simulink model "PoseEstimationController"  (R2017a)
settings: Solver=FixedStepDiscrete  StartTime=0.0  StopTime=10.0  RelTol=1e-3
values from neighbouring files (symbols this model uses):
  dt = dtFC    [evalOriginSensordata.m]    (also in startControllerNL.m = 0.01)
  H_Drone = zeros(5,12)    [evalOriginSensordata.m]    (also in startControllerNL.m)
  H_TWB = zeros(3,12)    [evalOriginSensordata.m]    (also in startControllerNL.m)
  k1 = a    (= 1)    [evalOriginSensordata.m]    (also in startControllerNL.m)
  k10 = a    (= 1)    [evalOriginSensordata.m]    (also in startControllerNL.m)
  k11 = a    (= 1)    [evalOriginSensordata.m]    (also in startControllerNL.m)
  k12 = a    (= 1)    [evalOriginSensordata.m]    (also in startControllerNL.m)
  k2 = a    (= 1)    [evalOriginSensordata.m]    (also in startControllerNL.m)
  k3 = a    (= 1)    [evalOriginSensordata.m]    (also in startControllerNL.m)
  k4 = a    (= 1)    [evalOriginSensordata.m]    (also in startControllerNL.m)
  k5 = a    (= 1)    [evalOriginSensordata.m]    (also in startControllerNL.m)
  k6 = a    (= 1)    [evalOriginSensordata.m]    (also in startControllerNL.m)
  k7 = a    (= 1)    [evalOriginSensordata.m]    (also in startControllerNL.m)
  k8 = a    (= 1)    [evalOriginSensordata.m]    (also in startControllerNL.m)
  k9 = a    (= 1)    [evalOriginSensordata.m]    (also in startControllerNL.m)
  kd1 = d    (= 10)    [evalOriginSensordata.m]    (also in startControllerNL.m)
  kd2 = d    (= 10)    [evalOriginSensordata.m]    (also in startControllerNL.m)
  kd3 = d    (= 10)    [evalOriginSensordata.m]    (also in startControllerNL.m)
  kd4 = d    (= 10)    [evalOriginSensordata.m]    (also in startControllerNL.m)
  kp1 = p    (= 5)    [evalOriginSensordata.m]    (also in startControllerNL.m)
  kp2 = p    (= 5)    [evalOriginSensordata.m]    (also in startControllerNL.m)
  kp3 = p    (= 5)    [evalOriginSensordata.m]    (also in startControllerNL.m)
  kp4 = p    (= 5)    [evalOriginSensordata.m]    (also in startControllerNL.m)
libraries: sharedTrackingLibrary x1
settings Model: Creator=Schalker  LastModifiedBy=Schalker
settings OptimizationCC: DefaultParameterBehavior=Inlined  UseDivisionForNetSlopeComputation=on  UseFloatMulNetSlope=on  InlineInvariantSignals=on  PassReuseOutputArgsAs=Individual arguments  ZeroExternalMemoryAtStartup=off  ZeroInternalMemoryAtStartup=off  NoFixptDivByZeroProtection=on  EfficientFloat2IntCast=on  LifeSpan=1  MaxStackSize=64
settings DebuggingCC: ParameterTunabilityLossMsg=error
settings HardwareCC: ProdBitPerPointer=32  ProdBitPerSizeT=32  ProdBitPerPtrDiffT=32  ProdLargestAtomicFloat=None  ProdWordSize=32  ProdHWDeviceType=Custom Processor->Custom
settings SFSimCC: MATLABDynamicMemAlloc=off
settings RTWCC: SystemTargetFile=ert.tlc  GenCodeOnly=on  TemplateMakefile=ert_default_tmf  Description=Embedded Coder  GenerateReport=on  Toolchain=Microsoft Visual C++ 2015 v14.0 | nmake (64-bit Windows)  IncludeHyperlinkInReport=on  LaunchReport=on  TargetLang=C++  GenerateTraceInfo=on  GenerateTraceReport=on  GenerateTraceReportSl=on  GenerateTraceReportSf=on  GenerateTraceReportEml=on  GenerateCodeMetricsReport=on
settings CodeAppCC: ForceParamTrailComments=on  IgnoreCustomStorageClasses=off  OperatorAnnotations=on  SimulinkDataObjDesc=on  SFDataObjDesc=on  MATLABFcnDesc=on  CustomSymbolStrGlobalVar=rt$N$M  CustomSymbolStrType=$N$M  CustomSymbolStrFcn=$N$M$F  CustomSymbolStrMacro=$N$M  InsertBlockDesc=on  MATLABSourceComments=on
settings ERTTargetCC: TargetLangStandard=C++03 (ISO)  IncludeMdlTerminateFcn=off  CombineSignalStateStructs=on  SupportAbsoluteTime=off  SupportComplex=off  SupportNonInlinedSFcns=on  InlinedParameterPlacement=NonHierarchical  RootIOFormat=Structure reference  ERTCustomFileTemplate=example_file_process.tlc  ERTFilePackagingFormat=CompactWithDataFile

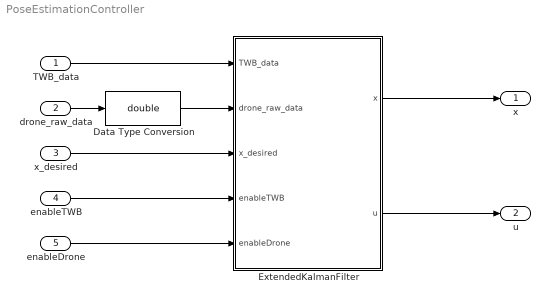
== system PoseEstimationController ==
  "TWB_data " : Inport  OutDataTypeStr=double  PortDimensions=3
  drone_raw_data : Inport  Port=2  OutDataTypeStr=uint8  PortDimensions=11
  x_desired : Inport  Port=3  OutDataTypeStr=double  PortDimensions=4
  enableTWB : Inport  Port=4  OutDataTypeStr=boolean  PortDimensions=1
  enableDrone : Inport  Port=5  OutDataTypeStr=boolean  PortDimensions=1
  Data Type Conversion : DataTypeConversion  OutDataTypeStr=double
  "ExtendedKalmanFilter " : Subsystem  InitFcn=|
      | t_end = 10;
      | Ts = 1/100; %0.05;
      | dt = 1/100;
      | 
      | k1 = 0.5;
      | k2 = 0.5;
      | k3 = 0.5;
      | k4 = 0.5;
      | k5 = 0.5;
      | k6 = 0.5;
      | k7 = 0.5;
      | k8 = 0.5;
      | k9 = 0.5;
      | k10 = 0.5;
      | k11 = 0.5;
      | k12 = 0.5;
      | 
      | a = 1;
      | k1 = a;
      | k2 = a;
      | k3 = a;
      | k4 = a;
      | k5 = a;
      | k6 = a;
      | k7 = a;
      | k8 = a;
      | k9 = a;
      | k10 = a;
      | k11 = a;
      | k12 = a;
      | 
      | p = 5;
      | kp1 = p;
      | kp2 = p;
      | kp3 = p;
      | kp4 = p;
      | 
      | d = 10;
      | kd1 = d;
      | kd2 = d;
      | kd3 = d;
      | kd4 = d;
      | 
      | processNoiseCovariance = eye(12,12)*0.5;
      | measurementNoiseCovarianceTWB = [0.000114037489420717 -2.82089891064414e-06 1.40417613824518e-05;-2.82089891064414e-06 0.000115657032079071 1.08946618253263e-06;1.40417613824518e-05 1.08946618253263e-06 0.00137780347424666];
      | measurementNoiseCovarianceDrone = [7.40493968128454e-07 4.00871171116695e-08 2.64850251168023e-07 4.81776544321576e-08 1.70610840898493e-07;4.00871171116695e-08 1.12410457478521e-06 -8.65404287048207e-08 -1.99569229909733e-07 2.12891815399967e-07;2.64850251168023e-07 -8.65404287048207e-08 3.89370394407336e-05 -1.56813743542319e-06 -2.34614557587901e-06;4.81776544321576e-08 -1.99569229909733e-07 -1.56813743542319e-06 3.83263259074627e-05 1.99513110891507e-06;1.70610840898493e-07 2.12891815399967e-07 -2.34614557587901e-06 1.99513110891507e-06 2.60130783647397e-05];
      | H_TWB = zeros(3,12);
      | H_TWB(1,1) = 1;
      | H_TWB(2,2) = 1;
      | H_TWB(3,3) = 1;
      | 
      | H_Drone = zeros(5,12);
      | H_Drone(1,7) = 1;
      | H_Drone(2,8) = 1;
      | H_Drone(3,9) = 1;
      | H_Drone(4,10) = 1;
      | H_Drone(5,11) = 1;
  x : Outport
  u : Outport  Port=2  OutDataTypeStr=uint8
  wires:
  drone_raw_data/1 -> Data Type Conversion/1
  x_desired/1 -> "ExtendedKalmanFilter "/3(x_desired)
  "ExtendedKalmanFilter "/1(x) -> x/1
  "ExtendedKalmanFilter "/2(u) -> u/1
  Data Type Conversion/1 -> "ExtendedKalmanFilter "/2(drone_raw_data)
  "TWB_data "/1 -> "ExtendedKalmanFilter "/1(TWB_data)
  enableTWB/1 -> "ExtendedKalmanFilter "/4(enableTWB)
  enableDrone/1 -> "ExtendedKalmanFilter "/5(enableDrone)

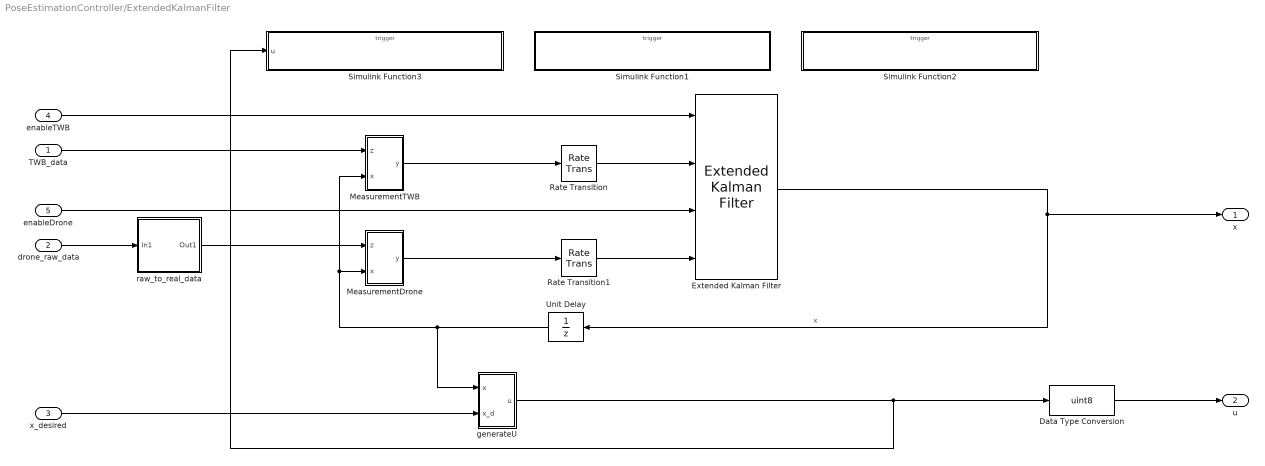
== system PoseEstimationController/ExtendedKalmanFilter  ==
  TWB_data : Inport
  drone_raw_data : Inport  Port=2
  x_desired : Inport  Port=3
  enableTWB : Inport  Port=4
  enableDrone : Inport  Port=5
  Data Type Conversion : DataTypeConversion  OutDataTypeStr=uint8
  Extended Kalman Filter : sharedTrackingLibrary/Extended Kalman Filter  StateTransitionFcn=stateTransitionFcn  HasStateTransitionJacobianFcn=off  HasAdditiveProcessNoise=Additive  ProcessNoise=processNoiseCovariance  HasTimeVaryingProcessNoise=off  HasStateTransitionFcnExtraArgument=0  InitialState=zeros(12, 1)  InitialStateCovariance=10  MeasurementFcn1=measurementTWBFcn  HasMeasurementJacobianFcn1=off  HasMeasurementEnablePort1=on  HasAdditiveMeasurementNoise1=Additive  MeasurementNoise1=measurementNoiseCovarianceTWB  HasTimeVaryingMeasurementNoise1=off  HasMeasurementFcnExtraArgument1=0  MeasurementFcn2=measurementDroneFcn  HasMeasurementJacobianFcn2=off  HasMeasurementEnablePort2=on  HasAdditiveMeasurementNoise2=Additive  MeasurementNoise2=measurementNoiseCovarianceDrone  HasTimeVaryingMeasurementNoise2=off  HasMeasurementFcnExtraArgument2=0  MeasurementFcn3=myMeasurementFcn  HasMeasurementJacobianFcn3=off  HasMeasurementEnablePort3=off  HasAdditiveMeasurementNoise3=Additive  MeasurementNoise3=1  HasTimeVaryingMeasurementNoise3=off  HasMeasurementFcnExtraArgument3=0  MeasurementFcn4=myMeasurementFcn  HasMeasurementJacobianFcn4=off  HasMeasurementEnablePort4=off  HasAdditiveMeasurementNoise4=Additive  MeasurementNoise4=1  HasTimeVaryingMeasurementNoise4=off  HasMeasurementFcnExtraArgument4=0  MeasurementFcn5=myMeasurementFcn  HasMeasurementJacobianFcn5=off  HasMeasurementEnablePort5=off  HasAdditiveMeasurementNoise5=Additive  MeasurementNoise5=1  HasTimeVaryingMeasurementNoise5=off  HasMeasurementFcnExtraArgument5=0  EnableMultirate=on  StateTransitionFcnSampleTime=dt  MeasurementFcn1SampleTime=dt  MeasurementFcn2SampleTime=dt  MeasurementFcn3SampleTime=1  MeasurementFcn4SampleTime=1  MeasurementFcn5SampleTime=1  UseCurrentEstimator=on  OutputStateCovariance=off  DataType=double  SampleTime=1  NumberOfMeasurements=2
  MeasurementDrone : Subsystem
  MeasurementTWB : Subsystem
  Rate Transition : RateTransition
  Rate Transition1 : RateTransition
  Simulink Function1 : Subsystem  TreatAsAtomicUnit=on
  Simulink Function2 : Subsystem  TreatAsAtomicUnit=on
  Simulink Function3 : Subsystem  TreatAsAtomicUnit=on
  Unit Delay : UnitDelay  SampleTime=-1
  generateU : Subsystem
  raw_to_real_data : Subsystem
  x : Outport
  u : Outport  Port=2
  wires:
  TWB_data/1 -> MeasurementTWB/1(z)
  x_desired/1 -> generateU/2("x_d ")
  Extended Kalman Filter/1 -> Unit Delay/1, x/1  "x"
  MeasurementDrone/1(y) -> Rate Transition1/1
  Rate Transition1/1 -> Extended Kalman Filter/4
  drone_raw_data/1 -> raw_to_real_data/1(In1)
  Rate Transition/1 -> Extended Kalman Filter/2
  Unit Delay/1 -> MeasurementDrone/2(x), MeasurementTWB/2(x), generateU/1(x)
  generateU/1(u) -> Data Type Conversion/1, Simulink Function3/1(u)
  MeasurementTWB/1(y) -> Rate Transition/1
  raw_to_real_data/1(Out1) -> MeasurementDrone/1(z)
  Data Type Conversion/1 -> u/1
  enableTWB/1 -> Extended Kalman Filter/1
  enableDrone/1 -> Extended Kalman Filter/3

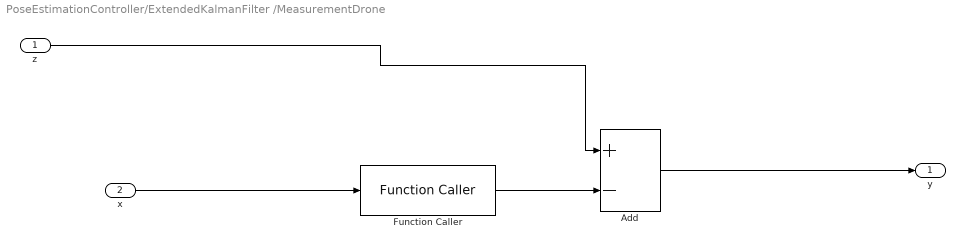
== system PoseEstimationController/ExtendedKalmanFilter /MeasurementDrone ==
  z : Inport
  x : Inport  Port=2
  Add : Sum  Inputs=+-
  Function Caller : FunctionCaller  FunctionPrototype=y = measurementDroneFcn(x)
  y : Outport
  wires:
  Add/1 -> y/1
  z/1 -> Add/1
  Function Caller/1 -> Add/2
  x/1 -> Function Caller/1

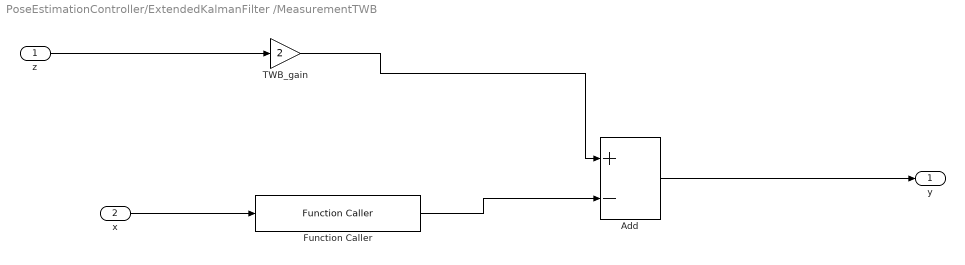
== system PoseEstimationController/ExtendedKalmanFilter /MeasurementTWB ==
  z : Inport
  x : Inport  Port=2
  Add : Sum  Inputs=+-
  Function Caller : FunctionCaller  FunctionPrototype=y = measurementTWBFcn(x)
  TWB_gain : Gain  Gain=2
  y : Outport
  wires:
  z/1 -> TWB_gain/1
  Add/1 -> y/1
  Function Caller/1 -> Add/2
  x/1 -> Function Caller/1
  TWB_gain/1 -> Add/1

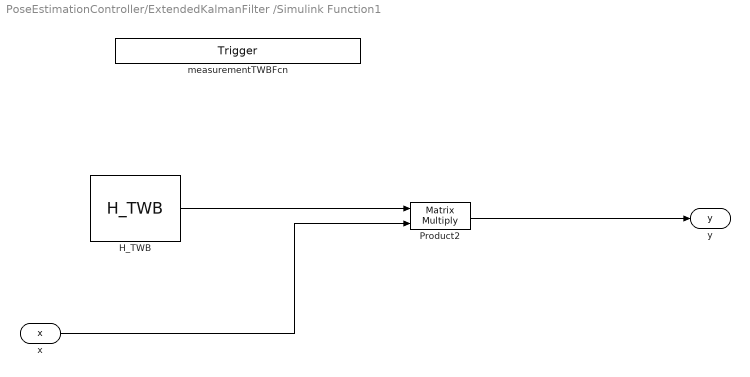
== system PoseEstimationController/ExtendedKalmanFilter /Simulink Function1 ==
  measurementTWBFcn : TriggerPort  TriggerType=function-call  IsSimulinkFunction=on  FunctionName=measurementTWBFcn  VariantControl=Variant
  H_TWB : Constant  Value=H_TWB
  Product2 : Product  Multiplication=Matrix(*)
  x : ArgIn  DisableCoverage=on  PortDimensions=12  ArgumentName=x
  y : ArgOut  DisableCoverage=on  PortDimensions=3  ArgumentName=y
  wires:
  H_TWB/1 -> Product2/1
  x/1 -> Product2/2
  Product2/1 -> y/1

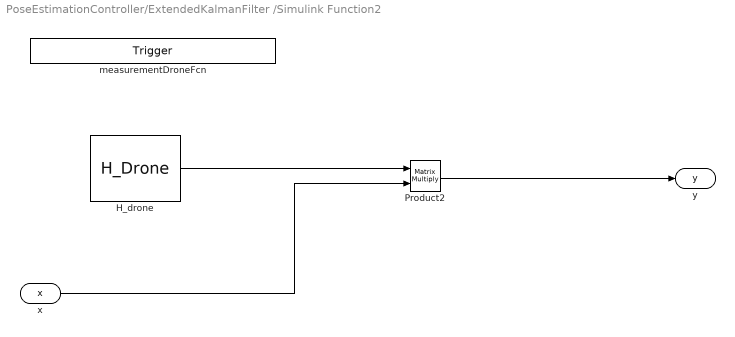
== system PoseEstimationController/ExtendedKalmanFilter /Simulink Function2 ==
  measurementDroneFcn : TriggerPort  TriggerType=function-call  IsSimulinkFunction=on  FunctionName=measurementDroneFcn  VariantControl=Variant
  H_drone : Constant  Value=H_Drone
  Product2 : Product  Multiplication=Matrix(*)
  x : ArgIn  DisableCoverage=on  PortDimensions=12  ArgumentName=x
  y : ArgOut  DisableCoverage=on  PortDimensions=5  ArgumentName=y
  wires:
  Product2/1 -> y/1
  H_drone/1 -> Product2/1
  x/1 -> Product2/2

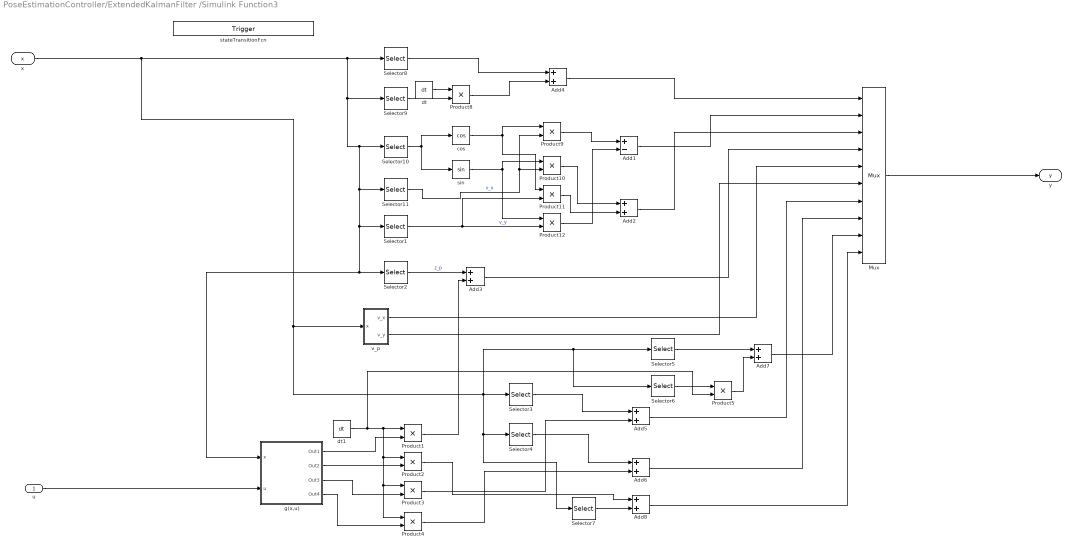
== system PoseEstimationController/ExtendedKalmanFilter /Simulink Function3 ==
  u : Inport
  stateTransitionFcn : TriggerPort  TriggerType=function-call  IsSimulinkFunction=on  FunctionName=stateTransitionFcn  VariantControl=Variant
  Add1 : Sum  Inputs=+-
  Add{2..8} (7 alike) : Sum
  Mux : Mux  Inputs=10
  Product{1..5,8..12} (10 alike) : Product
  Selector1 : Selector  InputPortWidth=12  IndexOptions=Index vector (dialog)  Indices=[8]  OutputSizes=1
  Selector10 : Selector  InputPortWidth=12  IndexOptions=Index vector (dialog)  Indices=[11]  OutputSizes=1
  Selector11 : Selector  InputPortWidth=12  IndexOptions=Index vector (dialog)  Indices=[7]  OutputSizes=1
  Selector2 : Selector  InputPortWidth=12  IndexOptions=Index vector (dialog)  Indices=[6]  OutputSizes=1
  Selector3 : Selector  InputPortWidth=12  IndexOptions=Index vector (dialog)  Indices=[9]  OutputSizes=1
  Selector4 : Selector  InputPortWidth=12  IndexOptions=Index vector (dialog)  Indices=[10]  OutputSizes=1
  Selector5 : Selector  InputPortWidth=12  IndexOptions=Index vector (dialog)  Indices=[11]  OutputSizes=1
  Selector6 : Selector  InputPortWidth=12  IndexOptions=Index vector (dialog)  Indices=[12]  OutputSizes=1
  Selector7 : Selector  InputPortWidth=12  IndexOptions=Index vector (dialog)  Indices=[12]  OutputSizes=1
  Selector8 : Selector  InputPortWidth=12  IndexOptions=Index vector (dialog)  Indices=[1 2 3]  OutputSizes=1
  Selector9 : Selector  InputPortWidth=12  IndexOptions=Index vector (dialog)  Indices=[4 5 6]  OutputSizes=1
  cos : Trigonometry  Operator=cos
  dt : Constant  Value=dt
  dt1 : Constant  Value=dt
  g(x,u) : Subsystem
  sin : Trigonometry
  v_p : Subsystem
  x : ArgIn  DisableCoverage=on  PortDimensions=12  ArgumentName=x
  y : ArgOut  DisableCoverage=on  PortDimensions=12  ArgumentName=y
  wires:
  x/1 -> Selector6/1, Selector5/1, Selector7/1, Selector4/1, Selector3/1, v_p/1(x), Selector8/1, Selector11/1, Selector1/1, Selector2/1, g(x,u)/1(x), Selector10/1, Selector9/1
  Selector9/1 -> Product8/2
  dt/1 -> Product8/1
  Product8/1 -> Add4/2
  Selector8/1 -> Add4/1
  Add4/1 -> Mux/1
  Selector10/1 -> sin/1, cos/1
  cos/1 -> Product11/1, Product9/1
  sin/1 -> Product12/1, Product10/1
  u/1 -> g(x,u)/2(u)
  Selector11/1 -> Product10/2, Product9/2  "v_x"
  Selector1/1 -> Product12/2, Product11/2  "v_y"
  Product9/1 -> Add1/1
  Product12/1 -> Add1/2
  Product10/1 -> Add2/1
  Product11/1 -> Add2/2
  Selector2/1 -> Add3/1  "z_p"
  g(x,u)/1(Out1) -> Product1/2
  Product1/1 -> Add3/2
  g(x,u)/2(Out2) -> Product2/2
  g(x,u)/3(Out3) -> Product3/2
  g(x,u)/4(Out4) -> Product4/2
  Add3/1 -> Mux/4
  v_p/1(v_x) -> Mux/5
  v_p/2(v_y) -> Mux/6
  Add1/1 -> Mux/2
  Add2/1 -> Mux/3
  Selector3/1 -> Add5/1
  Product3/1 -> Add5/2
  Selector4/1 -> Add6/1
  Product4/1 -> Add6/2
  Add5/1 -> Mux/7
  Add6/1 -> Mux/8
  Selector6/1 -> Product5/1
  dt1/1 -> Product5/2, Product2/1, Product4/1, Product3/1, Product1/1
  Selector5/1 -> Add7/1
  Product5/1 -> Add7/2
  Add7/1 -> Mux/9
  Selector7/1 -> Add8/2
  Product2/1 -> Add8/1
  Add8/1 -> Mux/10
  Mux/1 -> y/1

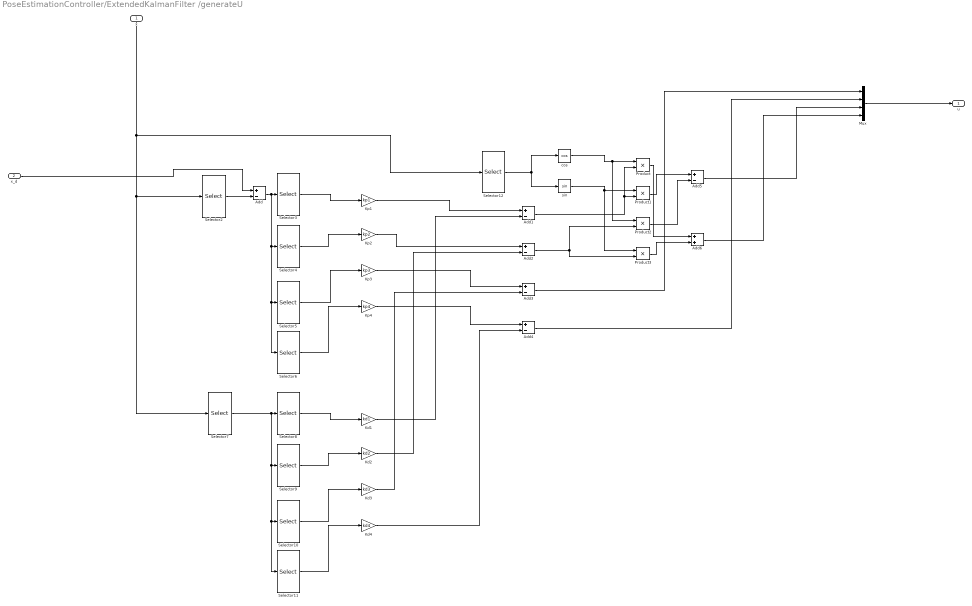
== system PoseEstimationController/ExtendedKalmanFilter /generateU ==
  x : Inport
  "x_d " : Inport  Port=2
  Add{,1..5} (6 alike) : Sum  Inputs=+-
  Add6 : Sum
  Kd1 : Gain  Gain=kd1
  Kd2 : Gain  Gain=kd2
  Kd3 : Gain  Gain=kd3
  Kd4 : Gain  Gain=kd4
  Kp1 : Gain  Gain=kp1
  Kp2 : Gain  Gain=kp2
  Kp3 : Gain  Gain=kp3
  Kp4 : Gain  Gain=kp4
  Mux : Mux
  Product{,1..3} (4 alike) : Product
  Selector10 : Selector  InputPortWidth=4  IndexOptions=Index vector (dialog)  Indices=3  OutputSizes=1
  Selector11 : Selector  InputPortWidth=4  IndexOptions=Index vector (dialog)  Indices=4  OutputSizes=1
  Selector12 : Selector  InputPortWidth=12  IndexOptions=Index vector (dialog)  Indices=11  OutputSizes=1
  Selector2 : Selector  InputPortWidth=12  IndexOptions=Index vector (dialog)  Indices=[1 2 3 11]  OutputSizes=1
  Selector3 : Selector  InputPortWidth=4  IndexOptions=Index vector (dialog)  Indices=[1]  OutputSizes=1
  Selector4 : Selector  InputPortWidth=4  IndexOptions=Index vector (dialog)  Indices=2  OutputSizes=1
  Selector5 : Selector  InputPortWidth=4  IndexOptions=Index vector (dialog)  Indices=3  OutputSizes=1
  Selector6 : Selector  InputPortWidth=4  IndexOptions=Index vector (dialog)  Indices=4  OutputSizes=1
  Selector7 : Selector  InputPortWidth=12  IndexOptions=Index vector (dialog)  Indices=[4 5 6 12]  OutputSizes=1
  Selector8 : Selector  InputPortWidth=4  IndexOptions=Index vector (dialog)  Indices=[1]  OutputSizes=1
  Selector9 : Selector  InputPortWidth=4  IndexOptions=Index vector (dialog)  Indices=2  OutputSizes=1
  cos : Trigonometry  Operator=cos
  sin : Trigonometry
  u : Outport
  wires:
  Selector3/1 -> Kp1/1
  "x_d "/1 -> Add/1
  Kp2/1 -> Add2/1
  Product2/1 -> Add5/2
  Add2/1 -> Product3/2, Product2/2
  Selector4/1 -> Kp2/1
  Add4/1 -> Mux/2
  Selector2/1 -> Add/2
  Add6/1 -> Mux/4
  Add5/1 -> Mux/3
  Product1/1 -> Add5/1
  Kp1/1 -> Add1/1
  Selector6/1 -> Kp4/1
  Kd4/1 -> Add4/2
  Add3/1 -> Mux/1
  Selector11/1 -> Kd4/1
  Selector7/1 -> Selector8/1, Selector9/1, Selector10/1, Selector11/1
  Selector10/1 -> Kd3/1
  Selector9/1 -> Kd2/1
  Selector8/1 -> Kd1/1
  Kd3/1 -> Add3/2
  Kp4/1 -> Add4/1
  Add1/1 -> Product1/2, Product/2
  Selector12/1 -> cos/1, sin/1
  Add/1 -> Selector6/1, Selector5/1, Selector4/1, Selector3/1
  Kd1/1 -> Add1/2
  x/1 -> Selector12/1, Selector7/1, Selector2/1
  Kp3/1 -> Add3/1
  Product3/1 -> Add6/2
  Product/1 -> Add6/1
  cos/1 -> Product2/1, Product/1
  sin/1 -> Product3/1, Product1/1
  Kd2/1 -> Add2/2
  Mux/1 -> u/1
  Selector5/1 -> Kp3/1

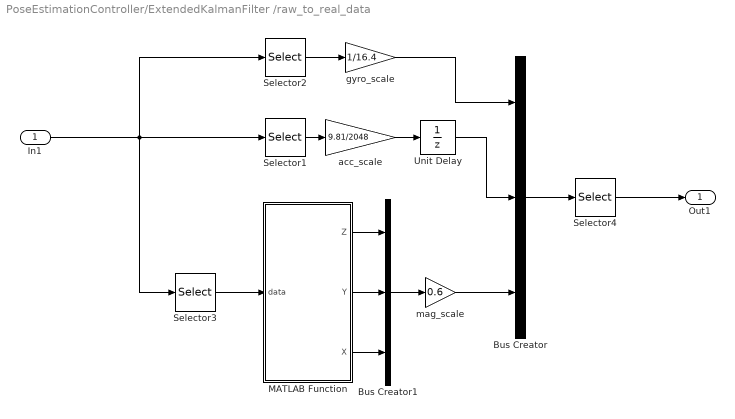
== system PoseEstimationController/ExtendedKalmanFilter /raw_to_real_data ==
  In1 : Inport  PortDimensions=11
  Bus Creator : BusCreator  Inputs=3
  Bus Creator1 : BusCreator  Inputs=3
  MATLAB Function : MATLAB Function  TreatAsAtomicUnit=on
  Selector1 : Selector  InputPortWidth=11  IndexOptions=Index vector (dialog)  Indices=[4,5,6]  OutputSizes=1
  Selector2 : Selector  InputPortWidth=11  IndexOptions=Index vector (dialog)  Indices=[1,2,3]  OutputSizes=1
  Selector3 : Selector  InputPortWidth=11  IndexOptions=Index vector (dialog)  Indices=[1:9]  OutputSizes=1
  Selector4 : Selector  InputPortWidth=9  IndexOptions=Index vector (dialog)  Indices=[4,5,7,8,9]  OutputSizes=1
  Unit Delay : UnitDelay  SampleTime=-1
  acc_scale : Gain  Gain=9.81/2048
  gyro_scale : Gain  Gain=1/16.4
  mag_scale : Gain  Gain=0.6
  Out1 : Outport  PortDimensions=5
  wires:
  In1/1 -> Selector3/1, Selector1/1, Selector2/1
  MATLAB Function/1(Z) -> Bus Creator1/1
  Bus Creator/1 -> Selector4/1
  Selector2/1 -> gyro_scale/1
  Selector1/1 -> acc_scale/1
  gyro_scale/1 -> Bus Creator/1
  Selector3/1 -> MATLAB Function/1(data)
  MATLAB Function/2(Y) -> Bus Creator1/2
  mag_scale/1 -> Bus Creator/3
  MATLAB Function/3(X) -> Bus Creator1/3
  Selector4/1 -> Out1/1
  Bus Creator1/1 -> mag_scale/1
  acc_scale/1 -> Unit Delay/1
  Unit Delay/1 -> Bus Creator/2

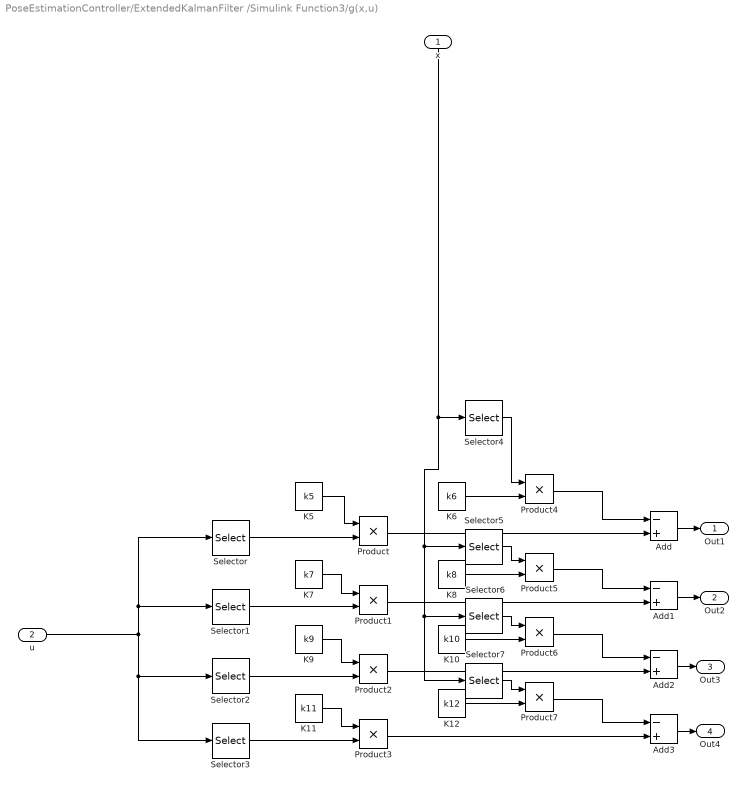
== system PoseEstimationController/ExtendedKalmanFilter /Simulink Function3/g(x,u) ==
  x : Inport
  u : Inport  Port=2
  Add{,1..3} (4 alike) : Sum  Inputs=-+
  K10 : Constant  Value=k10
  K11 : Constant  Value=k11
  K12 : Constant  Value=k12
  K5 : Constant  Value=k5
  K6 : Constant  Value=k6
  K7 : Constant  Value=k7
  K8 : Constant  Value=k8
  K9 : Constant  Value=k9
  Product{,1..7} (8 alike) : Product
  Selector : Selector  InputPortWidth=4  IndexOptions=Index vector (dialog)  Indices=[1]  OutputSizes=1
  Selector1 : Selector  InputPortWidth=4  IndexOptions=Index vector (dialog)  Indices=[2]  OutputSizes=1
  Selector2 : Selector  InputPortWidth=4  IndexOptions=Index vector (dialog)  Indices=[3]  OutputSizes=1
  Selector3 : Selector  InputPortWidth=4  IndexOptions=Index vector (dialog)  Indices=[4]  OutputSizes=1
  Selector4 : Selector  InputPortWidth=12  IndexOptions=Index vector (dialog)  Indices=[6]  OutputSizes=1
  Selector5 : Selector  InputPortWidth=12  IndexOptions=Index vector (dialog)  Indices=[12]  OutputSizes=1
  Selector6 : Selector  InputPortWidth=12  IndexOptions=Index vector (dialog)  Indices=[9]  OutputSizes=1
  Selector7 : Selector  InputPortWidth=12  IndexOptions=Index vector (dialog)  Indices=[10]  OutputSizes=1
  Out1 : Outport
  Out2 : Outport  Port=2
  Out3 : Outport  Port=3
  Out4 : Outport  Port=4
  wires:
  K7/1 -> Product1/1
  Selector6/1 -> Product6/1
  Selector2/1 -> Product2/2
  Product/1 -> Add/2
  Product6/1 -> Add2/1
  Selector/1 -> Product/2
  Add2/1 -> Out3/1
  x/1 -> Selector7/1, Selector6/1, Selector5/1, Selector4/1
  Add3/1 -> Out4/1
  Add/1 -> Out1/1
  Add1/1 -> Out2/1
  K9/1 -> Product2/1
  Selector4/1 -> Product4/1
  u/1 -> Selector/1, Selector1/1, Selector3/1, Selector2/1
  Product2/1 -> Add2/2
  K8/1 -> Product5/2
  Product3/1 -> Add3/2
  Product1/1 -> Add1/2
  Selector5/1 -> Product5/1
  Product5/1 -> Add1/1
  Selector3/1 -> Product3/2
  K5/1 -> Product/1
  K12/1 -> Product7/2
  Product7/1 -> Add3/1
  K10/1 -> Product6/2
  Product4/1 -> Add/1
  Selector1/1 -> Product1/2
  Selector7/1 -> Product7/1
  K11/1 -> Product3/1
  K6/1 -> Product4/2

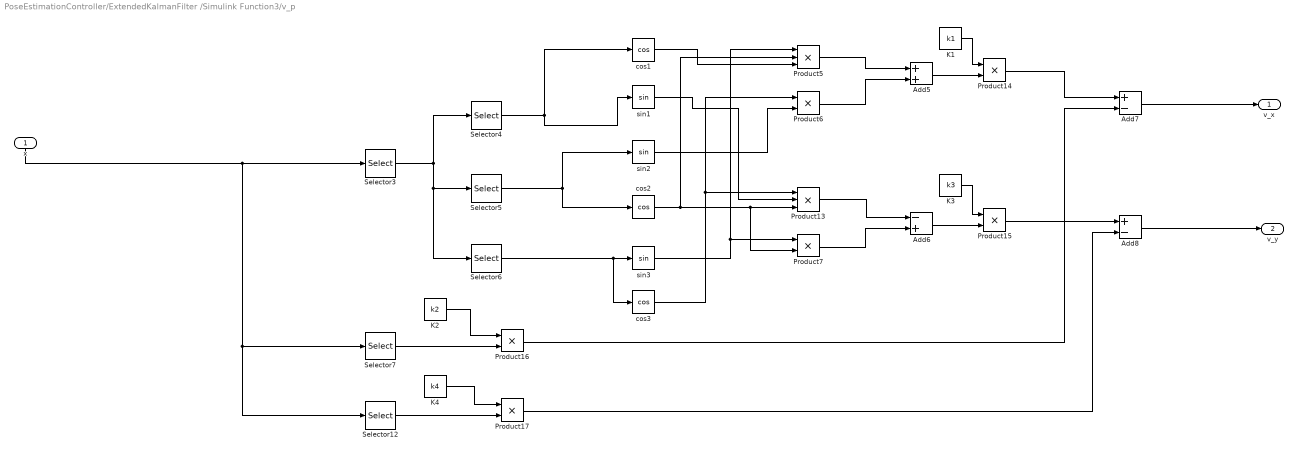
== system PoseEstimationController/ExtendedKalmanFilter /Simulink Function3/v_p ==
  x : Inport
  Add5 : Sum
  Add6 : Sum  Inputs=-+
  Add7 : Sum  Inputs=+-
  Add8 : Sum  Inputs=+-
  K1 : Constant  Value=k1
  K2 : Constant  Value=k2
  K3 : Constant  Value=k3
  K4 : Constant  Value=k4
  Product13 : Product  Inputs=3
  Product{6..7,14..17} (6 alike) : Product
  Product5 : Product  Inputs=3
  Selector12 : Selector  InputPortWidth=12  IndexOptions=Index vector (dialog)  Indices=[8]  OutputSizes=1
  Selector3 : Selector  InputPortWidth=12  IndexOptions=Index vector (dialog)  Indices=[9 10 11]  OutputSizes=1
  Selector4 : Selector  InputPortWidth=3  IndexOptions=Index vector (dialog)  Indices=[1]  OutputSizes=1
  Selector5 : Selector  InputPortWidth=3  IndexOptions=Index vector (dialog)  Indices=[2]  OutputSizes=1
  Selector6 : Selector  InputPortWidth=3  IndexOptions=Index vector (dialog)  Indices=[3]  OutputSizes=1
  Selector7 : Selector  InputPortWidth=12  IndexOptions=Index vector (dialog)  Indices=[7]  OutputSizes=1
  cos1 : Trigonometry  Operator=cos
  cos2 : Trigonometry  Operator=cos
  cos3 : Trigonometry  Operator=cos
  sin1 : Trigonometry
  sin2 : Trigonometry
  sin3 : Trigonometry
  v_x : Outport
  v_y : Outport  Port=2
  wires:
  x/1 -> Selector12/1, Selector7/1, Selector3/1
  Selector6/1 -> sin3/1, cos3/1
  sin2/1 -> Product6/2
  Product6/1 -> Add5/2
  Add7/1 -> v_x/1
  Add5/1 -> Product14/2
  K1/1 -> Product14/1
  Product13/1 -> Add6/1
  Product16/1 -> Add7/2
  Product17/1 -> Add8/2
  cos2/1 -> Product7/2, Product13/3, Product5/2
  K2/1 -> Product16/1
  Selector5/1 -> cos2/1, sin2/1
  sin1/1 -> Product13/2
  Add8/1 -> v_y/1
  Selector7/1 -> Product16/2
  Product14/1 -> Add7/1
  sin3/1 -> Product5/1, Product7/1
  Product5/1 -> Add5/1
  Selector12/1 -> Product17/2
  Selector4/1 -> cos1/1, sin1/1
  Selector3/1 -> Selector6/1, Selector5/1, Selector4/1
  Product7/1 -> Add6/2
  Product15/1 -> Add8/1
  Add6/1 -> Product15/2
  cos3/1 -> Product13/1, Product6/1
  cos1/1 -> Product5/3
  K4/1 -> Product17/1
  K3/1 -> Product15/1

== matlab function PoseEstimationController/ExtendedKalmanFilter /raw_to_real_data/MATLAB Function ==
  data: data input; Z output; Y output; X output
function [Z,Y,X] = fcn(data)
    %% Process sensor data through algorithm
    data = data';
    gyroscope = data(1,[1:3]);
    accelerometer = data(1,[4:6]);
    magnetometer = data(1,[7:9]);
    AHRS = MadgwickAHRS('SamplePeriod', 1/256, 'Beta', 0.1);
    % AHRS = MahonyAHRS('SamplePeriod', 1/256, 'Kp', 0.5);

    quaternion = zeros(1, 4);
    AHRS.Update(gyroscope(1,:) * (pi/180), accelerometer(1,:), magnetometer(1,:));	% gyroscope units must be radians
    quaternion = AHRS.Quaternion;

    euler = quatern2euler(quaternConj(quaternion)) * (180/pi);	% use conjugate for sensor frame relative to Earth and convert to degrees.
    Z = euler(1,1);
    Y = euler(1,2);
    X = euler(1,3);

end

% function obj = MadgwickAHRS(varargin)
%     for i = 1:2:nargin
%         if  strcmp(varargin{i}, 'SamplePeriod'), obj.SamplePeriod = varargin{i+1};
%         elseif  strcmp(varargin{i}, 'Quaternion'), obj.Quaternion = varargin{i+1};
%         elseif  strcmp(varargin{i}, 'Beta'), obj.Beta = varargin{i+1};
%         else error('Invalid argument');
%         end
%     end;
% end
% function obj = Update(obj, Gyroscope, Accelerometer, Magnetometer)
%     q = obj.Quaternion; % short name local variable for readability
% 
%     % Normalise accelerometer measurement
%     if(norm(Accelerometer) == 0), return; end	% handle NaN
%     Accelerometer = Accelerometer / norm(Accelerometer);	% normalise magnitude
% 
%     % Normalise magnetometer measurement
%     if(norm(Magnetometer) == 0), return; end	% handle NaN
%     Magnetometer = Magnetometer / norm(Magnetometer);	% normalise magnitude
% 
%     % Reference direction of Earth's magnetic feild
%     h = quaternProd(q, quaternProd([0 Magnetometer], quaternConj(q)));
%     b = [0 norm([h(2) h(3)]) 0 h(4)];
% 
%     % Gradient decent algorithm corrective step
%     F = [2*(q(2)*q(4) - q(1)*q(3)) - Accelerometer(1)
%         2*(q(1)*q(2) + q(3)*q(4)) - Accelerometer(2)
%         2*(0.5 - q(2)^2 - q(3)^2) - Accelerometer(3)
%         2*b(2)*(0.5 - q(3)^2 - q(4)^2) + 2*b(4)*(q(2)*q(4) - q(1)*q(3)) - Magnetometer(1)
%         2*b(2)*(q(2)*q(3) - q(1)*q(4)) + 2*b(4)*(q(1)*q(2) + q(3)*q(4)) - Magnetometer(2)
%         2*b(2)*(q(1)*q(3) + q(2)*q(4)) + 2*b(4)*(0.5 - q(2)^2 - q(3)^2) - Magnetometer(3)];
%     J = [-2*q(3),                 	2*q(4),                    -2*q(1),                         2*q(2)
%         2*q(2),                 	2*q(1),                    	2*q(4),                         2*q(3)
%         0,                         -4*q(2),                    -4*q(3),                         0
%         -2*b(4)*q(3),               2*b(4)*q(4),               -4*b(2)*q(3)-2*b(4)*q(1),       -4*b(2)*q(4)+2*b(4)*q(2)
%         -2*b(2)*q(4)+2*b(4)*q(2),	2*b(2)*q(3)+2*b(4)*q(1),	2*b(2)*q(2)+2*b(4)*q(4),       -2*b(2)*q(1)+2*b(4)*q(3)
%         2*b(2)*q(3),                2*b(2)*q(4)-4*b(4)*q(2),	2*b(2)*q(1)-4*b(4)*q(3),        2*b(2)*q(2)];
%     step = (J'*F);
%     step = step / norm(step);	% normalise step magnitude
% 
%     % Compute rate of change of quaternion
%     qDot = 0.5 * quaternProd(q, [0 Gyroscope(1) Gyroscope(2) Gyroscope(3)]) - obj.Beta * step';
% 
%     % Integrate to yield quaternion
%     q = q + qDot * obj.SamplePeriod;
%     obj.Quaternion = q / norm(q); % normalise quaternion
% end
% 
% function obj = UpdateIMU(obj, Gyroscope, Accelerometer)
%     q = obj.Quaternion; % short name local variable for readability
% 
%     % Normalise accelerometer measurement
%     if(norm(Accelerometer) == 0), return; end	% handle NaN
%     Accelerometer = Accelerometer / norm(Accelerometer);	% normalise magnitude
% 
%     % Gradient decent algorithm corrective step
%     F = [2*(q(2)*q(4) - q(1)*q(3)) - Accelerometer(1)
%         2*(q(1)*q(2) + q(3)*q(4)) - Accelerometer(2)
%         2*(0.5 - q(2)^2 - q(3)^2) - Accelerometer(3)];
%     J = [-2*q(3),	2*q(4),    -2*q(1),	2*q(2)
%         2*q(2),     2*q(1),     2*q(4),	2*q(3)
%         0,         -4*q(2),    -4*q(3),	0    ];
%     step = (J'*F);
%     step = step / norm(step);	% normalise step magnitude
% 
%     % Compute rate of change of quaternion
%     qDot = 0.5 * quaternProd(q, [0 Gyroscope(1) Gyroscope(2) Gyroscope(3)]) - obj.Beta * step';
% 
%     % Integrate to yield quaternion
%     q = q + qDot * obj.SamplePeriod;
%     obj.Quaternion = q / norm(q); % normalise quaternion
% end
